simulink model "track"  (R2019a)
settings: Solver=VariableStepAuto  StartTime=0.0  StopTime=50  FixedStep=0.01  RelTol=1e-3
values from neighbouring files (symbols this model uses):
  g = 9.8    [grasp_test.m]    (also in my_mpc.m; track_test.m; xz2dof_para.m)
  Ixx = 3*0.114    (= 0.342)    [my_mpc.m]    (also in track_test.m; xz2dof_para.m)
  Iyy = 3*0.114    (= 0.342)    [my_mpc.m]    (also in track_test.m; xz2dof_para.m)
  Izz = 3*0.158    (= 0.474)    [my_mpc.m]    (also in track_test.m; xz2dof_para.m)
  kati = 3e-4    (= 0.0003)    [track_test.m]
  katp = 5    [track_test.m]
  kctd = 1    [track_test.m]
  kcti = 3e-4    (= 0.0003)    [track_test.m]
  kctp = 5    [track_test.m]
  kdp = 4000    [track_test.m]
  kdph = 4000    [track_test.m]
  kdt = 4000    [track_test.m]
  kdx = 0.8    [track_test.m]    (also in xz2dof_para.m = 17)
  kdy = 0.8    [track_test.m]
  kdz = 1.5    [track_test.m]    (also in xz2dof_para.m = 50)
  Kf = 6.11e-8*3600/4/pi^2    (= 5.57165188849e-06)    [track_test.m]
  kix = 0    [track_test.m]    (also in xz2dof_para.m = 10)
  kiy = 0    [track_test.m]
  kiz = 0    [track_test.m]    (also in xz2dof_para.m)
  Km = 1.5e-9*3600/4/pi^2    (= 1.36783597917e-07)    [track_test.m]
  km = 20    [track_test.m]
  kpp = 800    [track_test.m]
  kpph = 2000    [track_test.m]
  kpt = 2000    [track_test.m]
  kpx = 1    [track_test.m]    (also in xz2dof_para.m = 180)
  kpy = 1    [track_test.m]
  kpz = 1.8    [track_test.m]    (also in xz2dof_para.m = 50)
  L = factorial(l)/factorial(l-4)    [getQ.m]    (also in my_mpc.m = 0.3; track_test.m = 0.3; xz2dof_para.m = 0.3)
  ms = mb+mL1+mL2    (= 1.78)    [my_mpc.m]    (also in track_test.m = 1.96; xz2dof_para.m = 1.96)
  pdes = [0 0 0;0 0 4;4 0 4;4 4 4]    [track_test.m]
  pointnum = length(pdes)-2    [track_test.m]
  psides = 0    [track_test.m]
  vdes = 2    [track_test.m]
  wh = sqrt(ms*g/4/Kf)    [track_test.m]
  xdes = final(1)    [track_test.m]
  ydes = final(2)    [track_test.m]
  zdes = final(3)    [track_test.m]
libraries: dspindex x2, shared6dof x1
settings Model: Creator=Administrator  LastModifiedBy=Administrator
settings DataIOCC: ReturnWorkspaceOutputs=off

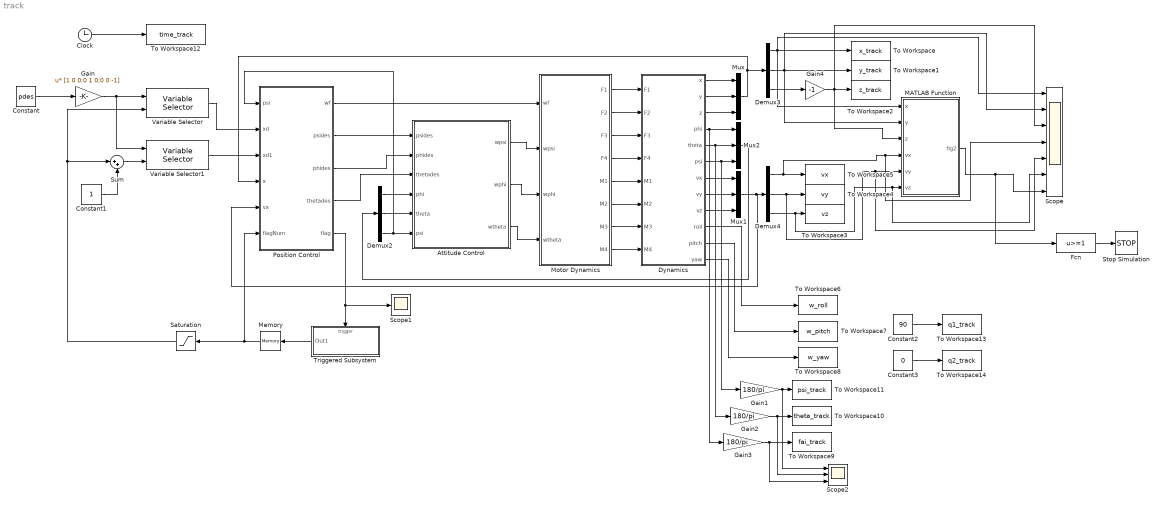
== system track ==
  Attitude Control : Subsystem
  Clock : Clock
  Constant : Constant  Value=pdes
  Constant1 : Constant
  Constant2 : Constant  Value=90
  Constant3 : Constant  Value=0
  Demux2 : Demux  Outputs=3
  Demux3 : Demux  Outputs=3
  Demux4 : Demux  Outputs=3
  Dynamics : Subsystem
  Fcn : Fcn  Expr=u>=1
  Gain : Gain  Gain=[1 0 0;0 1 0;0 0 -1]  Multiplication=Matrix(u*K)
  Gain1 : Gain  Gain=180/pi
  Gain2 : Gain  Gain=180/pi
  Gain3 : Gain  Gain=180/pi
  Gain4 : Gain  Gain=-1
  MATLAB Function : MATLAB Function  TreatAsAtomicUnit=on
  Memory : Memory
  Motor Dynamics : Subsystem
  Mux : Mux  Inputs=3
  Mux1 : Mux  Inputs=3
  Mux2 : Mux  Inputs=3
  Position Control : Subsystem
  Saturation : Saturate  UpperLimit=pointnum  LowerLimit=0
  Scope : Scope  NumInputPorts=7
  Scope1 : Scope
  Scope2 : Scope  NumInputPorts=3
  Stop Simulation : Stop
  Sum : Sum  Inputs=|++
  To Workspace : ToWorkspace  VariableName=x_track  SampleTime=-1
  To Workspace1 : ToWorkspace  VariableName=y_track  SampleTime=-1
  To Workspace10 : ToWorkspace  VariableName=theta_track  SampleTime=-1
  To Workspace11 : ToWorkspace  VariableName=psi_track  SampleTime=-1
  To Workspace12 : ToWorkspace  VariableName=time_track  SampleTime=-1
  To Workspace13 : ToWorkspace  VariableName=q1_track  SampleTime=-1
  To Workspace14 : ToWorkspace  VariableName=q2_track  SampleTime=-1
  To Workspace2 : ToWorkspace  VariableName=z_track  SampleTime=-1
  To Workspace3 : ToWorkspace  VariableName=vz  SampleTime=-1
  To Workspace4 : ToWorkspace  VariableName=vy  SampleTime=-1
  To Workspace5 : ToWorkspace  VariableName=vx  SampleTime=-1
  To Workspace6 : ToWorkspace  VariableName=w_roll  SampleTime=-1
  To Workspace7 : ToWorkspace  VariableName=w_pitch  SampleTime=-1
  To Workspace8 : ToWorkspace  VariableName=w_yaw  SampleTime=-1
  To Workspace9 : ToWorkspace  VariableName=fai_track  SampleTime=-1
  Triggered Subsystem : Subsystem  TreatAsAtomicUnit=on
  Variable Selector : dspindex/Variable Selector  NumInputs=1  rowsOrCols=Rows  IdxMode=Variable  Elements=[1 3]  ZerOneIdxMode=Zero-based  errmode=Clip Index  FillMode=on  FillValues=0
  Variable Selector1 : dspindex/Variable Selector  NumInputs=1  rowsOrCols=Rows  IdxMode=Variable  Elements=[1 3]  ZerOneIdxMode=Zero-based  errmode=Clip Index  FillMode=on  FillValues=0
  wires:
  Motor Dynamics/4(F4) -> Dynamics/4(F4)
  Motor Dynamics/6(M2) -> Dynamics/6(M2)
  Demux3/3 -> Gain4/1
  Gain3/1 -> Scope2/3, To Workspace9/1
  Gain4/1 -> MATLAB Function/3(z), Scope/3, To Workspace2/1
  Position Control/1(wf) -> Motor Dynamics/1(wf)
  Motor Dynamics/2(F2) -> Dynamics/2(F2)
  Demux3/1 -> MATLAB Function/1(x), Scope/1, To Workspace/1
  Gain1/1 -> Scope2/1, To Workspace11/1
  Gain2/1 -> Scope2/2, To Workspace10/1
  Demux3/2 -> MATLAB Function/2(y), Scope/2, To Workspace1/1
  Dynamics/4(phi) -> Mux2/1, Gain3/1
  Dynamics/5(theta) -> Mux2/2, Gain2/1
  Dynamics/12(yaw) -> To Workspace8/1
  Dynamics/3(z) -> Mux/3
  Gain/1 -> Variable Selector1/1, Variable Selector/1
  Dynamics/10(roll) -> To Workspace6/1
  Dynamics/11(pitch) -> To Workspace7/1
  Demux4/1 -> Scope/4, MATLAB Function/4(vx), To Workspace5/1
  Dynamics/2(y) -> Mux/2
  Dynamics/1(x) -> Mux/1
  Dynamics/9(vz) -> Mux1/3
  Dynamics/8(vy) -> Mux1/2
  Motor Dynamics/7(M3) -> Dynamics/7(M3)
  Motor Dynamics/8(M4) -> Dynamics/8(M4)
  Motor Dynamics/5(M1) -> Dynamics/5(M1)
  Motor Dynamics/3(F3) -> Dynamics/3(F3)
  Memory/1 -> Saturation/1, Position Control/6(flagNum)
  Position Control/2(psides) -> Attitude Control/1(psides)
  Motor Dynamics/1(F1) -> Dynamics/1(F1)
  Attitude Control/2(wphi) -> Motor Dynamics/3(wphi)
  Attitude Control/3(wtheta) -> Motor Dynamics/4(wtheta)
  Attitude Control/1(wpsi) -> Motor Dynamics/2(wpsi)
  Constant1/1 -> Sum/2
  Triggered Subsystem/1(Out1) -> Memory/1
  Position Control/5(flag) -> Scope1/1, Triggered Subsystem/Trigger
  Variable Selector1/1 -> Position Control/3(xd1)
  Variable Selector/1 -> Position Control/2(xd)
  Demux4/3 -> Scope/6, MATLAB Function/6(vz), To Workspace3/1
  Demux4/2 -> Scope/5, MATLAB Function/5(vy), To Workspace4/1
  Mux2/1 -> Demux2/1
  Sum/1 -> Variable Selector1/2
  Demux2/2 -> Attitude Control/5(theta)
  Demux2/3 -> Position Control/1(psi), Attitude Control/6(psi)
  Demux2/1 -> Attitude Control/4(phi)
  Dynamics/7(vx) -> Mux1/1
  Mux1/1 -> Position Control/5(vx), Demux4/1
  Position Control/4(thetades) -> Attitude Control/3(thetades)
  Mux/1 -> Demux3/1, Position Control/4(x)
  Position Control/3(phides) -> Attitude Control/2(phides)
  Dynamics/6(psi) -> Mux2/3, Gain1/1
  MATLAB Function/1(flg2) -> Fcn/1, Scope/7
  Fcn/1 -> Stop Simulation/1
  Clock/1 -> To Workspace12/1
  Constant2/1 -> To Workspace13/1
  Constant3/1 -> To Workspace14/1
  Constant/1 -> Gain/1
  Saturation/1 -> Variable Selector/2, Sum/1

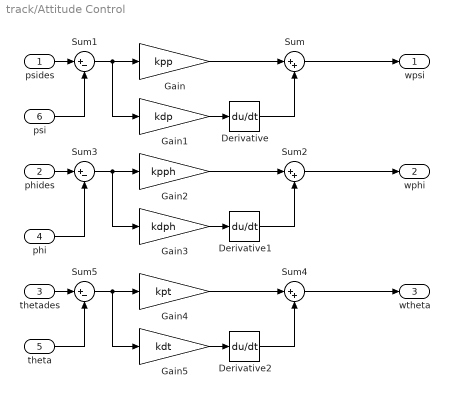
== system track/Attitude Control ==
  psides : Inport
  phides : Inport  Port=2
  thetades : Inport  Port=3
  phi : Inport  Port=4
  theta : Inport  Port=5
  psi : Inport  Port=6
  Derivative : Derivative
  Derivative1 : Derivative
  Derivative2 : Derivative
  Gain : Gain  Gain=kpp
  Gain1 : Gain  Gain=kdp
  Gain2 : Gain  Gain=kpph
  Gain3 : Gain  Gain=kdph
  Gain4 : Gain  Gain=kpt
  Gain5 : Gain  Gain=kdt
  Sum : Sum  Inputs=|++
  Sum1 : Sum  Inputs=|+-
  Sum2 : Sum  Inputs=|++
  Sum3 : Sum  Inputs=|+-
  Sum4 : Sum  Inputs=|++
  Sum5 : Sum  Inputs=|+-
  wpsi : Outport
  wphi : Outport  Port=2
  wtheta : Outport  Port=3
  wires:
  Gain1/1 -> Derivative/1
  Derivative/1 -> Sum/2
  Gain/1 -> Sum/1
  Sum/1 -> wpsi/1
  Sum1/1 -> Gain1/1, Gain/1
  psides/1 -> Sum1/1
  psi/1 -> Sum1/2
  Gain3/1 -> Derivative1/1
  Sum3/1 -> Gain3/1, Gain2/1
  phi/1 -> Sum3/2
  Gain2/1 -> Sum2/1
  phides/1 -> Sum3/1
  Derivative1/1 -> Sum2/2
  Sum2/1 -> wphi/1
  Gain5/1 -> Derivative2/1
  Sum5/1 -> Gain5/1, Gain4/1
  theta/1 -> Sum5/2
  Gain4/1 -> Sum4/1
  thetades/1 -> Sum5/1
  Derivative2/1 -> Sum4/2
  Sum4/1 -> wtheta/1

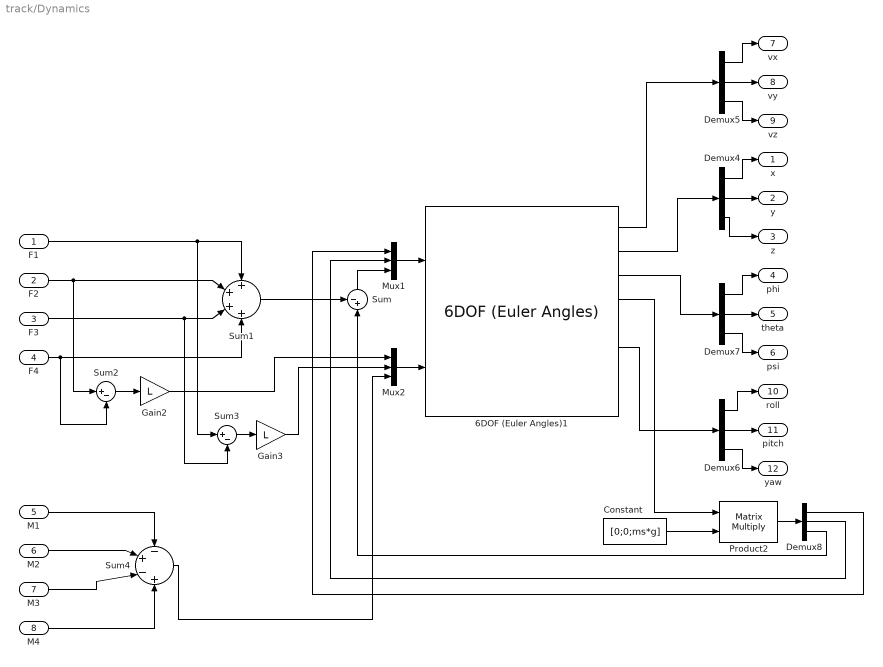
== system track/Dynamics ==
  F1 : Inport
  F2 : Inport  Port=2
  F3 : Inport  Port=3
  F4 : Inport  Port=4
  M1 : Inport  Port=5
  M2 : Inport  Port=6
  M3 : Inport  Port=7
  M4 : Inport  Port=8
  6DOF (Euler Angles)1 : shared6dof/6DOF (Euler Angles)  units=Metric (MKS)  mtype=Fixed  rep=Euler Angles  xme_0=[0 0 0]  Vm_0=[0 0 0]  eul_0=[0 0 0]  pm_0=[0 0 0]  mass_0=ms  mass_e=0.5  mass_f=2.0  inertia=[Ixx+0.08 0 0;0 Iyy+0.08 0;0 0 Izz+0.02]  inertia_e=eye(3)  inertia_f=2*eye(3)  k_quat=1.0  vre_flag=on  abi_flag=off  aMode=0  xme_statename=''  Vm_statename=''  eul_statename=''  quat_statename=''  pm_statename=''  mass_statename=''
      settings: SourceProductBaseCode=AE
  Constant : Constant  Value=[0;0;ms*g]
  Demux{4..8} (5 alike) : Demux  Outputs=3
  Gain2 : Gain  Gain=L
  Gain3 : Gain  Gain=L
  Mux1 : Mux  Inputs=3
  Mux2 : Mux  Inputs=3
  Product2 : Product  Multiplication=Matrix(*)
  Sum : Sum  Inputs=-+|
  Sum1 : Sum  Inputs=+|+|+|+
  Sum2 : Sum  Inputs=|+-
  Sum3 : Sum  Inputs=|+-
  Sum4 : Sum  Inputs=-|+|-|+
  x : Outport
  y : Outport  Port=2
  z : Outport  Port=3
  phi : Outport  Port=4
  theta : Outport  Port=5
  psi : Outport  Port=6
  vx : Outport  Port=7
  vy : Outport  Port=8
  vz : Outport  Port=9
  roll : Outport  Port=10
  pitch : Outport  Port=11
  yaw : Outport  Port=12
  wires:
  M3/1 -> Sum4/3
  M2/1 -> Sum4/2
  Sum2/1 -> Gain2/1
  M1/1 -> Sum4/1
  M4/1 -> Sum4/4
  Demux6/1 -> roll/1
  Demux6/2 -> pitch/1
  6DOF (Euler Angles)1/6 -> Demux6/1
  6DOF (Euler Angles)1/2 -> Demux4/1
  Demux4/2 -> y/1
  Demux5/2 -> vy/1
  Demux6/3 -> yaw/1
  Demux5/3 -> vz/1
  6DOF (Euler Angles)1/1 -> Demux5/1
  Demux4/1 -> x/1
  Demux5/1 -> vx/1
  Product2/1 -> Demux8/1
  6DOF (Euler Angles)1/4 -> Product2/1
  Demux7/3 -> psi/1
  Sum/1 -> Mux1/3
  Demux7/2 -> theta/1
  Demux8/1 -> Mux1/1
  Gain3/1 -> Mux2/2
  Sum4/1 -> Mux2/3
  F4/1 -> Sum2/2, Sum1/4
  F3/1 -> Sum3/2, Sum1/3
  Mux2/1 -> 6DOF (Euler Angles)1/2
  Demux7/1 -> phi/1
  Sum3/1 -> Gain3/1
  Constant/1 -> Product2/2
  6DOF (Euler Angles)1/3 -> Demux7/1
  Sum1/1 -> Sum/1
  Gain2/1 -> Mux2/1
  Demux8/3 -> Sum/2
  Demux8/2 -> Mux1/2
  F1/1 -> Sum3/1, Sum1/1
  F2/1 -> Sum2/1, Sum1/2
  Mux1/1 -> 6DOF (Euler Angles)1/1
  Demux4/3 -> z/1

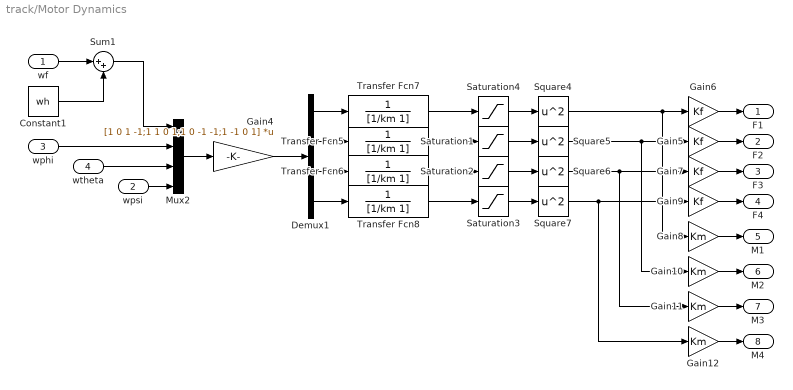
== system track/Motor Dynamics ==
  wf : Inport
  wpsi : Inport  Port=2
  wphi : Inport  Port=3
  wtheta : Inport  Port=4
  Constant1 : Constant  Value=wh
  Demux1 : Demux
  Gain{8,10..12} (4 alike) : Gain  Gain=Km
  Gain4 : Gain  Gain=[1 0 1 -1;1 1 0 1;1 0 -1 -1;1 -1 0 1]  Multiplication=Matrix(K*u) (u vector)
  Gain{5..7,9} (4 alike) : Gain  Gain=Kf
  Mux2 : Mux
  Saturation{1..4} (4 alike) : Saturate  UpperLimit=3*260*pi  LowerLimit=3*40*pi  ZeroCross=off
  Square{4..7} (4 alike) : Math  Operator=square  SaturateOnIntegerOverflow=on
  Sum1 : Sum  Inputs=|++
  Transfer Fcn{5..8} (4 alike) : TransferFcn  Denominator=[1/km 1]
  F1 : Outport
  F2 : Outport  Port=2
  F3 : Outport  Port=3
  F4 : Outport  Port=4
  M1 : Outport  Port=5
  M2 : Outport  Port=6
  M3 : Outport  Port=7
  M4 : Outport  Port=8
  wires:
  Gain6/1 -> F1/1
  wpsi/1 -> Mux2/4
  Demux1/4 -> Transfer Fcn8/1
  Demux1/1 -> Transfer Fcn7/1
  Gain4/1 -> Demux1/1
  Mux2/1 -> Gain4/1
  wphi/1 -> Mux2/2
  wtheta/1 -> Mux2/3
  Sum1/1 -> Mux2/1
  wf/1 -> Sum1/1
  Gain7/1 -> F3/1
  Square7/1 -> Gain12/1, Gain9/1
  Demux1/2 -> Transfer Fcn5/1
  Square6/1 -> Gain11/1, Gain7/1
  Demux1/3 -> Transfer Fcn6/1
  Gain9/1 -> F4/1
  Square5/1 -> Gain10/1, Gain5/1
  Gain10/1 -> M2/1
  Gain11/1 -> M3/1
  Gain8/1 -> M1/1
  Gain5/1 -> F2/1
  Gain12/1 -> M4/1
  Square4/1 -> Gain8/1, Gain6/1
  Constant1/1 -> Sum1/2
  Transfer Fcn7/1 -> Saturation4/1
  Saturation4/1 -> Square4/1
  Saturation1/1 -> Square5/1
  Transfer Fcn5/1 -> Saturation1/1
  Saturation2/1 -> Square6/1
  Transfer Fcn6/1 -> Saturation2/1
  Saturation3/1 -> Square7/1
  Transfer Fcn8/1 -> Saturation3/1

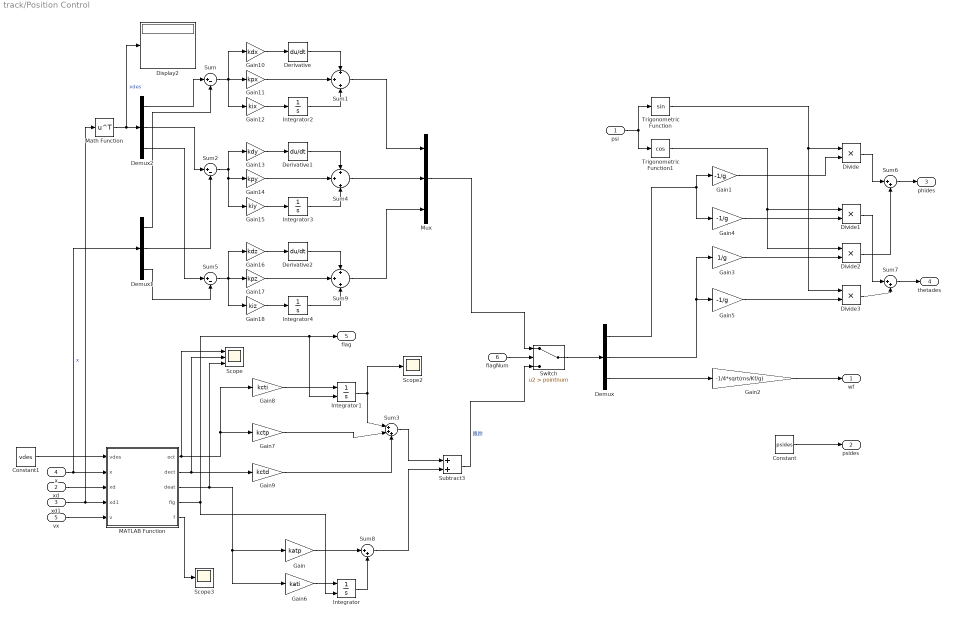
== system track/Position Control ==
  psi : Inport
  xd : Inport  Port=2
  xd1 : Inport  Port=3
  x : Inport  Port=4
  vx : Inport  Port=5
  flagNum : Inport  Port=6
  Constant : Constant  Value=psides
  Constant1 : Constant  Value=vdes
  Demux : Demux  Outputs=3
  Demux1 : Demux  Outputs=3
  Demux2 : Demux  Outputs=3
  Derivative : Derivative
  Derivative1 : Derivative
  Derivative2 : Derivative
  Display2 : Display
  Divide{,1..3} (4 alike) : Product  Inputs=**
  Gain : Gain  Gain=katp
  Gain1 : Gain  Gain=-1/g
  Gain10 : Gain  Gain=kdx
  Gain11 : Gain  Gain=kpx
  Gain12 : Gain  Gain=kix
  Gain13 : Gain  Gain=kdy
  Gain14 : Gain  Gain=kpy
  Gain15 : Gain  Gain=kiy
  Gain16 : Gain  Gain=kdz
  Gain17 : Gain  Gain=kpz
  Gain18 : Gain  Gain=kiz
  Gain2 : Gain  Gain=-1/4*sqrt(ms/Kf/g)
  Gain3 : Gain  Gain=1/g
  Gain4 : Gain  Gain=-1/g
  Gain5 : Gain  Gain=-1/g
  Gain6 : Gain  Gain=kati
  Gain7 : Gain  Gain=kctp
  Gain8 : Gain  Gain=kcti
  Gain9 : Gain  Gain=kctd
  Integrator : Integrator  ExternalReset=rising
  Integrator1 : Integrator  ExternalReset=rising
  Integrator2 : Integrator
  Integrator3 : Integrator
  Integrator4 : Integrator
  MATLAB Function : MATLAB Function  TreatAsAtomicUnit=on
  Math Function : Math  Operator=transpose  SaturateOnIntegerOverflow=on
  Mux : Mux  Inputs=3
  Scope : Scope  NumInputPorts=3
  Scope2 : Scope
  Scope3 : Scope
  Subtract3 : Sum
  Sum : Sum  Inputs=|+-
  Sum1 : Sum  Inputs=+|+|+
  Sum2 : Sum  Inputs=|+-
  Sum3 : Sum  Inputs=|+++
  Sum4 : Sum  Inputs=+|+|+
  Sum5 : Sum  Inputs=|+-
  Sum6 : Sum  Inputs=|++
  Sum7 : Sum  Inputs=|++
  Sum8 : Sum  Inputs=|++
  Sum9 : Sum  Inputs=+|+|+
  Switch : Switch  Criteria=u2 > Threshold  Threshold=pointnum
  Trigonometric Function : Trigonometry
  Trigonometric Function1 : Trigonometry  Operator=cos
  wf : Outport
  psides : Outport  Port=2
  phides : Outport  Port=3
  thetades : Outport  Port=4
  flag : Outport  Port=5
  wires:
  Demux/2 -> Gain3/1, Gain5/1
  Demux/1 -> Gain1/1, Gain4/1
  Demux/3 -> Gain2/1
  Gain2/1 -> wf/1
  Sum6/1 -> phides/1
  Sum7/1 -> thetades/1
  Constant/1 -> psides/1
  psi/1 -> Trigonometric Function1/1, Trigonometric Function/1
  Gain1/1 -> Divide/2
  Trigonometric Function/1 -> Divide3/1, Divide/1
  Divide/1 -> Sum6/1
  Trigonometric Function1/1 -> Divide2/1, Divide1/1
  Gain4/1 -> Divide1/2
  Divide1/1 -> Sum7/1
  Gain3/1 -> Divide2/2
  Divide2/1 -> Sum6/2
  Divide3/1 -> Sum7/2
  Gain5/1 -> Divide3/2
  Constant1/1 -> MATLAB Function/1(vdes)
  Gain6/1 -> Integrator/1
  Gain/1 -> Sum8/1
  Integrator/1 -> Sum8/2
  Gain8/1 -> Integrator1/1
  Gain7/1 -> Sum3/2
  Integrator1/1 -> Scope2/1, Sum3/1
  Gain9/1 -> Sum3/3
  Subtract3/1 -> Switch/3  "跟踪"
  Sum3/1 -> Subtract3/1
  Sum8/1 -> Subtract3/2
  MATLAB Function/1(ect) -> Scope/1, Gain7/1, Gain8/1
  MATLAB Function/2(dect) -> Scope/2, Gain9/1
  MATLAB Function/3(deat) -> Scope/3, Gain6/1, Gain/1
  MATLAB Function/4(flg) -> Integrator/2, Integrator1/2, flag/1
  x/1 -> Demux1/1, MATLAB Function/2(x)  "x"
  xd/1 -> MATLAB Function/3(xd)
  xd1/1 -> Math Function/1, MATLAB Function/4(xd1)
  vx/1 -> MATLAB Function/5(v)
  MATLAB Function/5(f) -> Scope3/1
  Math Function/1 -> Display2/1, Demux2/1  "xdes"
  Demux2/1 -> Sum/1
  Demux1/1 -> Sum/2
  Sum/1 -> Gain12/1, Gain11/1, Gain10/1
  Gain10/1 -> Derivative/1
  Gain12/1 -> Integrator2/1
  Gain11/1 -> Sum1/2
  Derivative/1 -> Sum1/1
  Integrator2/1 -> Sum1/3
  Sum2/1 -> Gain15/1, Gain14/1, Gain13/1
  Gain15/1 -> Integrator3/1
  Gain13/1 -> Derivative1/1
  Derivative1/1 -> Sum4/1
  Gain14/1 -> Sum4/2
  Integrator3/1 -> Sum4/3
  Sum5/1 -> Gain18/1, Gain17/1, Gain16/1
  Gain18/1 -> Integrator4/1
  Gain16/1 -> Derivative2/1
  Derivative2/1 -> Sum9/1
  Gain17/1 -> Sum9/2
  Integrator4/1 -> Sum9/3
  Demux2/2 -> Sum2/1
  Demux1/2 -> Sum2/2
  Demux2/3 -> Sum5/1
  Demux1/3 -> Sum5/2
  Sum1/1 -> Mux/1
  Sum4/1 -> Mux/2
  Sum9/1 -> Mux/3
  Mux/1 -> Switch/1
  Switch/1 -> Demux/1
  flagNum/1 -> Switch/2

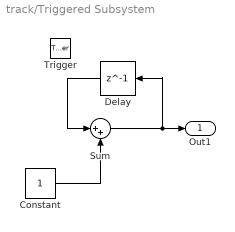
== system track/Triggered Subsystem ==
  Trigger : TriggerPort  VariantControl=Variant
  Constant : Constant
  Delay : Delay  DelayLength=1
  Sum : Sum  Inputs=|++
  Out1 : Outport
  wires:
  Sum/1 -> Delay/1, Out1/1
  Constant/1 -> Sum/2
  Delay/1 -> Sum/1

== matlab function track/Position Control/MATLAB Function ==
  data: vdes input; ect output; x input; xd input; xd1 input; v input; dect output; deat output; flg output; f output
function [ect,dect,deat,flg,f] = fcn(vdes,x,xd,xd1,v)
xd=xd';
xd1=xd1';
ti=xd1-xd;
abst=sqrt(sum(ti.^2));
ti=ti./abst;
ect=sum((x-xd).*ti)*ti-(x-xd);
dect=sum(v.*ti)*ti-v;
deat=vdes*ti-sum(v.*ti)*ti;
f=sum((x-xd1).*ti);
if f<0
    flg=0;
else
    flg=1;
end
end

== matlab function track/MATLAB Function ==
  data: x input; y input; z input; flg2 output; xdes parameter; ydes parameter; zdes parameter; vx input; vy input; vz input
function flg2 = fcn(x, y, z, xdes, ydes, zdes, vx, vy, vz)
    if (abs(x-xdes)<0.01) && (abs(y-ydes)<0.01) && abs(z-zdes)<0.01 && (abs(vx)<0.001) && (abs(vy)<0.001) && (abs(vz)<0.001)
        flg2 = 1;
    else
        flg2 = 0;
    end
end
